simulink model "lab6model"  (R2023a)
settings: Solver=ode45  StartTime=0.0  StopTime=0.5  MaxStep=0.001  RelTol=1e-3
values from neighbouring files (symbols this model uses):
  K = 18    [lab6main.m]    (also in lab6report.m)
  K_amp = 2.4    [lab6main.m]    (also in lab6report.m)
  K_c = 2    [lab6main.m]    (also in lab6report.m)
  K_pot = 10/2/pi    (= 1.59154943092)    [lab6main.m]    (also in lab6report.m)
  lower = -10    [lab6main.m]
  tau_m = 2/10    (= 0.2)    [lab6main.m]    (also in lab6report.m)
  tau_p = 0.0073    [lab6main.m]    (also in lab6report.m = 0.007)
  tau_z = 0.068    [lab6main.m]    (also in lab6report.m = 0.07)
  upper = 10    [lab6main.m]
  V_i = 50    [lab6main.m]
settings Model: Creator=rar4  LastModifiedBy=rar4

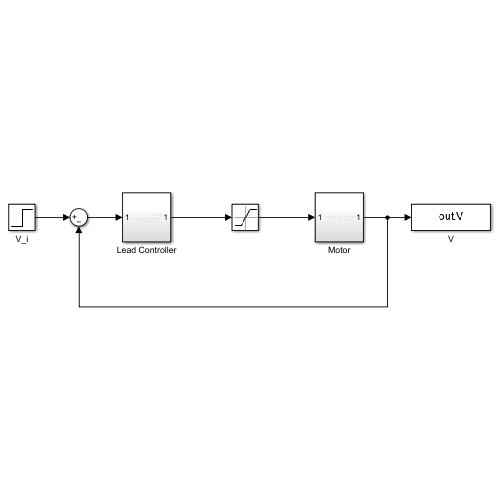
[thumbnail: Simulink's stored preview of the top-level diagram]
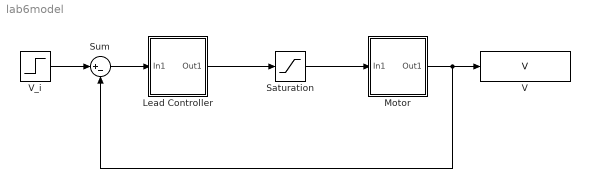
== system lab6model ==
  Lead Controller : Subsystem
  Motor : Subsystem
  Saturation : Saturate  UpperLimit=upper  LowerLimit=lower
  Sum : Sum  Inputs=|+-
  V : ToWorkspace  VariableName=V  SampleTime=-1
  V_i : Step  Time=0  After=V_i  SampleTime=0
  wires:
  V_i/1 -> Sum/1
  Sum/1 -> Lead Controller/1(In1)
  Lead Controller/1(Out1) -> Saturation/1
  Motor/1(Out1) -> Sum/2, V/1
  Saturation/1 -> Motor/1(In1)

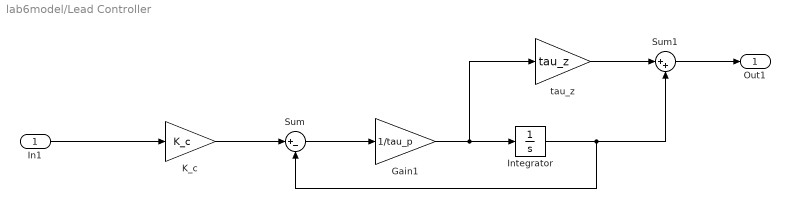
== system lab6model/Lead Controller ==
  In1 : Inport
  Gain1 : Gain  Gain=1/tau_p
  Integrator : Integrator
  K_c : Gain  Gain=K_c
  Sum : Sum  Inputs=|+-
  Sum1 : Sum  Inputs=|++
  tau_z : Gain  Gain=tau_z
  Out1 : Outport
  wires:
  K_c/1 -> Sum/1
  Sum/1 -> Gain1/1
  In1/1 -> K_c/1
  Gain1/1 -> tau_z/1, Integrator/1
  Integrator/1 -> Sum1/2, Sum/2
  tau_z/1 -> Sum1/1
  Sum1/1 -> Out1/1

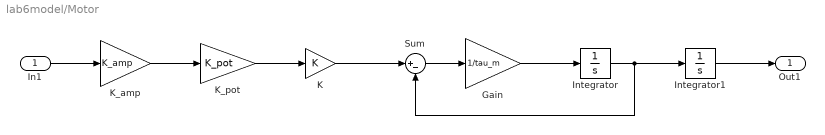
== system lab6model/Motor ==
  In1 : Inport
  Gain : Gain  Gain=1/tau_m
  Integrator : Integrator
  Integrator1 : Integrator
  K : Gain  Gain=K
  K_amp : Gain  Gain=K_amp
  K_pot : Gain  Gain=K_pot
  Sum : Sum  Inputs=|+-
  Out1 : Outport
  wires:
  K_pot/1 -> K/1
  K_amp/1 -> K_pot/1
  In1/1 -> K_amp/1
  K/1 -> Sum/1
  Sum/1 -> Gain/1
  Gain/1 -> Integrator/1
  Integrator/1 -> Sum/2, Integrator1/1
  Integrator1/1 -> Out1/1
